simulink model "sim_trajectory_tracking_template"  (R2024b)
settings: Solver=VariableStepAuto  StartTime=0.0  StopTime=T_SIM  MaxStep=0.001  RelTol=1e-3
undefined symbols (not defined in the file): control_par, controller_index, d, d_actual, omega_M, Q_INIT, r, r_actual, T_trj, trj_index
settings Model: Creator=alber  LastModifiedBy=alber
settings RTWCC: GPUComputeCapability=3.5

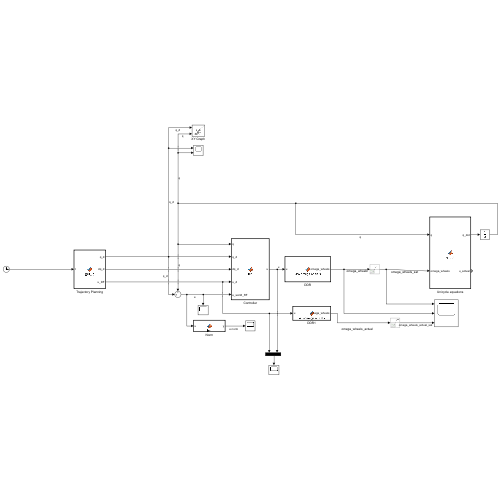
[thumbnail: Simulink's stored preview of the top-level diagram]
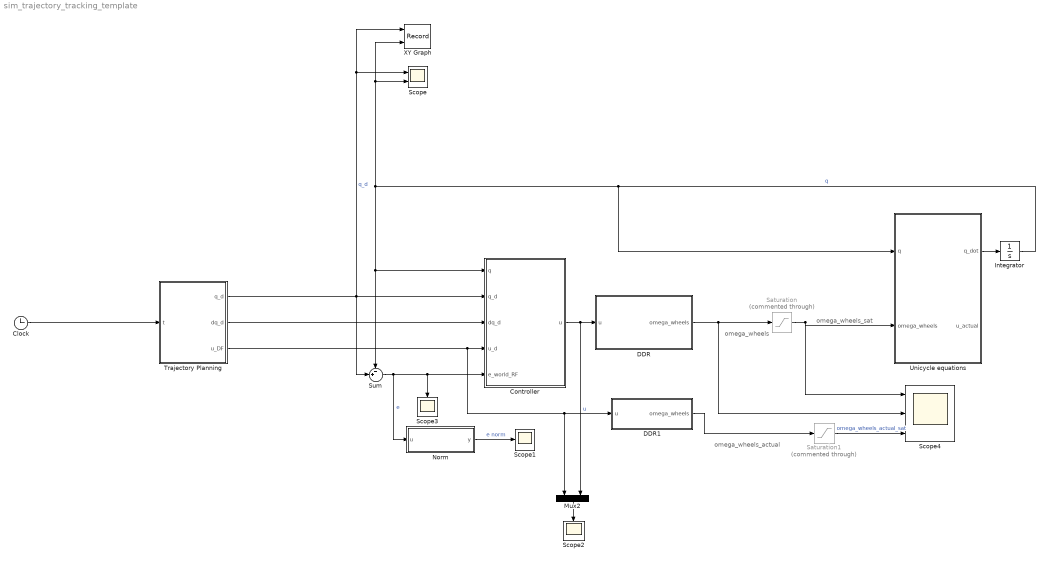
== system sim_trajectory_tracking_template ==
  note: omega_wheels_actual
  note: omega_wheels_sat
  note: omega_wheels
  Clock : Clock
  Controller : MATLAB Function  TreatAsAtomicUnit=on
  DDR : MATLAB Function  TreatAsAtomicUnit=on
  DDR1 : MATLAB Function  TreatAsAtomicUnit=on
  Integrator : Integrator  InitialCondition=Q_INIT
  Mux2 : Mux  Inputs=2
  Norm : MATLAB Function  TreatAsAtomicUnit=on
  Saturation : Saturate  Commented=through  UpperLimit=omega_M  LowerLimit=-omega_M
  Saturation1 : Saturate  Commented=through  UpperLimit=omega_M  LowerLimit=-omega_M
  Scope : Scope  NumInputPorts=2
  Scope1 : Scope
  Scope2 : Scope
  Scope3 : Scope
  Scope4 : Scope  NumInputPorts=3
  Sum : Sum  Inputs=-+|
  Trajectory Planning : MATLAB Function  TreatAsAtomicUnit=on
  Unicycle equations : MATLAB Function  TreatAsAtomicUnit=on
  XY Graph : Record  FileSettingsInternal="{\"entries\":[{\"content\":{\"excelSettings\":{\"content\":{},\"type\":\"Streamout.ExcelSettings\"}},\"type\":\"Streamout.FileSettingStorage\",\"uuid\":\"\"}],\"packageUris\":[\"http:\\/\\/schema.mathworks.com\\/mf0\\/streamout_blocks\\/R2020a\"],\"version\":\"1.0\"}"  Layout=[1 1]  SignalsInternal="{\"entries\":[{\"content\":{\"signals\":[{\"content\":{\"blockPath\":[],\"dimensions\":[3,1],\"domain\":\"\",\"hasChildren\":true,\"lineColor\":\"#fe330a\",\"port\":1,\"signalID\":1,\"signalName\":\"q_d\"},\"type\":\"RecordBlkView.Signal\",\"uuid\":\"\"},{\"content\":{\"blockPath\":[],\"channel\":[1,1],\"dimensions\":[3,1],\"domain\":\"\",\"lineColor\":\"#0072bd\",\"parentID\":1,\"plots\":[ 1 ],\"port\":1,\"signalID\":2,\"signalName\":\"q_d\"},\"type\":\"RecordBlkView.Signal\",\"uuid\":\"\"},{\"content\":{\"blockPath\":[],\"channel\":[2,1],\"dimensions\":[3,1],\"domain\":\"\",\"lineColor\":\"#0072bd\",\"parentID\":1,\"plots\":[ 1 ],\"port\":1,\"signalID\":3,\"signalName\":\"q_d\"},\"type\":\"RecordBlkView.Signal\",\"uuid\":\"\"},{\"content\":{\"blockPath\":[],\"channel\":[3,1],\"dimensions\":[3,1],\"domain\":\"\",\"lineColor\":\"#139fff\",\"parentID\":1,\"port\":1,\"signalID\":4,\"signalName\":\"q_d\"},\"type\":\"RecordBlkView.Signal\",\"uuid\":\"\"},{\"content\":{\"blockPath\":[],\"dimensions\":[3,1],\"domain\":\"\",\"hasChildren\":true,\"lineColor\":\"#0072bd\",\"port\":2,\"signalID\":5,\"signalName\":\"q\"},\"type\":\"RecordBlkView.Signal\",\"uuid\":\"\"},{\"content\":{\"blockPath\":[],\"channel\":[1,1],\"dimensions\":[3,1],\"domain\":\"\",\"lineColor\":\"#000000\",\"lineStyle\":\"DASH_DOT\",\"parentID\":5,\"plots\":[ 1 ],\"port\":2,\"signalID\":6,\"signalName\":\"q\"},\"type\":\"RecordBlkView.Signal\",\"uuid\":\"\"},{\"content\":{\"blockPath\":[],\"channel\":[2,1],\"dimensions\":[3,1],\"domain\":\"\",\"lineColor\":\"#000000\",\"lineStyle\":\"DASH_DOT\",\"parentID\":5,\"plots\":[ 1 ],\"port\":2,\"signalID\":7,\"signalName\":\"q\"},\"type\":\"RecordBlkView.Signal\",\"uuid\":\"\"},{\"content\":{\"blockPath\":[],\"channel\":[3,1],\"dimensions\":[3,1],\"domain\":\"\",\"lineColor\":\"#b746ff\",\"parentID\":5,\"port\":2,\"signalID\":8,\"signalName\":\"q\"},\"type\":\"RecordBlkView.Signal\",\"uuid\":\"\"}]},\"type\":\"RecordBlkView.InputSignals\",\"uuid\":\"\"}],\"packageUris\":[\"http:\\/\\/schema.mathworks.com\\/mf0\\/streamout_blocks\\/R2020a\"],\"version\":\"1.0\"}"  VisualizationBindings="{\"xyplotplugin\":{\"info\":[{\"series\":[{\"bindingParametersList\":[{\"parameter\":\"X-Axis\",\"signalID\":2,\"signalName\":\"q_d(1,1)\"},{\"parameter\":\"Y-Axis\",\"signalID\":3,\"signalName\":\"q_d(2,1)\"}],\"seriesID\":0},{\"bindingParametersList\":[{\"parameter\":\"X-Axis\",\"signalID\":6,\"signalName\":\"q(1,1)\"},{\"parameter\":\"Y-Axis\",\"signalID\":7,\"signalName\":\"q(2,1)\"}],\"seriesID\":1}],\"subplotID\":1}]}}"  CompatibilityTag=XY
  wires:
  Clock/1 -> Trajectory Planning/1(t)
  Integrator/1 -> Sum/1, Controller/1(q), Scope/2, XY Graph/2, Unicycle equations/1(q)  "q"
  Unicycle equations/1(q_dot) -> Integrator/1
  Trajectory Planning/1(q_d) -> Scope/1, XY Graph/1, Controller/2(q_d), Sum/2  "q_d"
  Sum/1 -> Norm/1(u), Controller/5(e_world_RF), Scope3/1  "e"
  Trajectory Planning/3(u_DF) -> Mux2/1, DDR1/1(u), Controller/4(u_d)
  Controller/1(u) -> DDR/1(u), Mux2/2  "u"
  Mux2/1 -> Scope2/1
  Trajectory Planning/2(dq_d) -> Controller/3(dq_d)
  Norm/1(y) -> Scope1/1  "e norm"
  DDR/1(omega_wheels) -> Saturation/1, Scope4/2
  Saturation/1 -> Scope4/1, Unicycle equations/2(omega_wheels)
  DDR1/1(omega_wheels) -> Saturation1/1
  Saturation1/1 -> Scope4/3  "omega_wheels_actual_sat"

== matlab function sim_trajectory_tracking_template/Norm ==
  data: u input; y output
function y = fcn(u)

y = sqrt(sum(u(1:2).^2));

== matlab function sim_trajectory_tracking_template/Unicycle equations ==
  data: q input; omega_wheels input; q_dot output; r_actual parameter; d_actual parameter; u_actual output
function [q_dot, u_actual] = q_dot(q, omega_wheels, r_actual, d_actual)
u_actual = [r_actual/2, r_actual/2;-r_actual/d_actual, r_actual/d_actual]*omega_wheels;
theta = q(3);
q_dot = [[cos(theta), 0];[sin(theta), 0];[0,1]]*u_actual;

== matlab function sim_trajectory_tracking_template/Trajectory Planning ==
  data: t input; q_d output; dq_d output; u_DF output; trj_index parameter; T_trj parameter
function [q_d, dq_d, u_DF] = get_trj(t, trj_index, T_trj)
if trj_index == 1
    % line
    vel = 1/T_trj;
    q_d = [0; vel*t; pi/2];
    dq_d = [0; vel; 0];
    u_DF = [vel; 0];
elseif trj_index == 2
    % circle
    r = 0.5;
    omega = 2*pi/T_trj;
    theta_prime = omega*t;
    q_d = [r*cos(theta_prime); r*sin(theta_prime); theta_prime + pi/2];
    dq_d = [-omega*r*sin(theta_prime); omega*r*cos(theta_prime); omega];
    u_DF = [omega*r; omega];
elseif trj_index == 3
    %  square
    T_cycle = mod(t, T_trj);
    side_length = 1;
    vel = side_length/(T_trj/4);
    if T_cycle<=T_trj/4
        t_side = T_cycle;
        q_d = [0;  t_side*vel; pi/2];
        dq_d = [0;vel;0];
        u_DF = [vel; 0];
    elseif T_cycle <=T_trj/2
        t_side = T_cycle - T_trj/4;
        q_d = [-vel*t_side; side_length ;pi];
        dq_d = [-vel;0;0];
        u_DF = [vel;0];
    elseif T_cycle <= 3*T_trj/4
        t_side = T_cycle - T_trj/2;
        q_d = [-side_length; side_length-vel*t_side; -pi/2];
        dq_d = [0;-vel;0];
        u_DF = [vel;0];
    else
        t_side = T_cycle - 3*T_trj/4;
        q_d = [-side_length + vel*t_side; 0; 0];
        dq_d = [vel;0;0];
        u_DF = [vel;0];
    end
elseif trj_index == 4
    % 8-shape
    R = 0.4;
    omega = 2*pi/T_trj;
    x_d = R*sin(2*omega*t);
    dx_d = R*2*omega*cos(2*omega*t);
    ddx_d = -R*4*omega.^2*sin(2*omega*t);
    y_d = R*sin(omega*t);
    dy_d = R*omega*cos(omega*t);
    ddy_d = -R*omega.^2*sin(omega*t);
    theta_d = atan2(dy_d, dx_d);
    dtheta_d = (dx_d*ddy_d -  dy_d*ddx_d)/(dx_d.^2+dy_d.^2);
    q_d = [x_d;y_d;theta_d];
    dq_d = [dx_d;dy_d;dtheta_d];
    u_DF = [sqrt(dx_d.^2 + dy_d.^2);dtheta_d];
else
    q_d = [0;0;0];
    dq_d = [0;0;0];
    u_DF = [0;0];
end

== matlab function sim_trajectory_tracking_template/Controller ==
  data: q input; q_d input; dq_d input; u_d input; u output; e_world_RF input; controller_index parameter; control_par parameter
function u = fcn(q, q_d, dq_d, u_d, e_world_RF, controller_index, control_par)
% compute the error in the unicycle RF
if controller_index == 1
    % linear controller
    u = u_d;
elseif controller_index == 2
    % nonlinear controller
    u = u_d;
elseif controller_index == 3
    % feedback linearization
    u = u_d;
else
    u = u_d;
end

== matlab function sim_trajectory_tracking_template/DDR ==
  data: u input; omega_wheels output; r parameter; d parameter
function omega_wheels = kin2omegawheels(u, r, d)
omega_l = u(1)/r-d/(2*r)*u(2);
omega_r = u(1)/r+d/(2*r)*u(2);
omega_wheels = [omega_l;omega_r];

== matlab function sim_trajectory_tracking_template/DDR1 ==
  data: u input; omega_wheels output; r_actual parameter; d_actual parameter
function omega_wheels = kin2omegawheels(u, r_actual, d_actual)
omega_l = u(1)/r_actual-d_actual/(2*r_actual)*u(2);
omega_r = u(1)/r_actual+d_actual/(2*r_actual)*u(2);
omega_wheels = [omega_l;omega_r];
